simulink model "ex7"  (Simulink 6.0)
settings: Solver=ode45  StartTime=0.0  StopTime=50000  RelTol=1e-3
values from neighbouring files (symbols this model uses):
  SymbolRate = 1000    [ex11.m]    (also in ex2sim.m = 2; ex4sim.m = 2; ex7sim.m = 2)
libraries: commutil2 x4, commsink2 x2, commdigbbndpm2 x2, commchan2 x1, commrandsrc2 x1
settings Model: LastModifiedBy=lxy

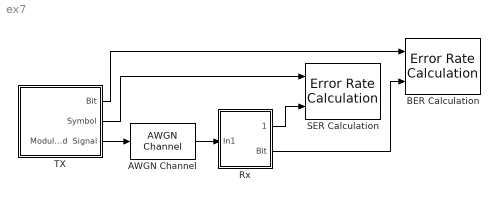
== system ex7 ==
  AWGN Channel : commchan2/AWGN Channel  seed=1111  noiseMode="Signal to noise ratio  (Es/No)"  EbNodB=10  EsNodB=SNR  SNRdB=10  bitsPerSym=1  Ps=1  Tsym=1/SymbolRate  variance=1
  BER Calculation : commsink2/Error Rate Calculation  N=0  st_delay=2*SymbolRate  cp_mode=Entire frame  subframe=[]  PMode=Workspace  WsName=BER  RsMode2=off  stop=on  numErr=100  maxBits=1e6
  Rx : Subsystem
  SER Calculation : commsink2/Error Rate Calculation  N=0  st_delay=SymbolRate  cp_mode=Entire frame  subframe=[]  PMode=Workspace  WsName=SER  RsMode2=off  stop=off  numErr=100  maxBits=1e6
  TX : Subsystem
  wires:
  TX/3(Modulated  Signal) -> AWGN Channel/1
  TX/2(Symbol) -> SER Calculation/1
  Rx/1(Symbol) -> SER Calculation/2
  Rx/2(Bit) -> BER Calculation/2
  TX/1(Bit) -> BER Calculation/1
  AWGN Channel/1 -> Rx/1(In1)

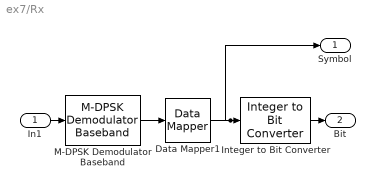
== system ex7/Rx ==
  In1 : Inport  Port=1  LatchInput=off
  Data Mapper1 : commutil2/Data Mapper  MapMode=Gray to Binary  M=4  MapVec=[0 1 3 2 7 6 4 5]
  Integer to Bit Converter : commutil2/Integer to Bit Converter  nbits=2
  M-DPSK Demodulator Baseband : commdigbbndpm2/M-DPSK Demodulator Baseband  M=4  OutType=Integer  Dec=Binary  Ph=0  numSamp=1
  Symbol : Outport
  Bit : Outport  Port=2
  wires:
  Integer to Bit Converter/1 -> Bit/1
  Data Mapper1/1 -> Symbol/1, Integer to Bit Converter/1
  In1/1 -> M-DPSK Demodulator Baseband/1
  M-DPSK Demodulator Baseband/1 -> Data Mapper1/1

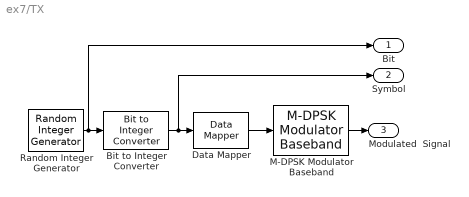
== system ex7/TX ==
  Bit to Integer Converter : commutil2/Bit to Integer Converter  nbits=2
  Data Mapper : commutil2/Data Mapper  MapMode=Binary to Gray  M=4  MapVec=[0 1 3 2 7 6 4 5]
  M-DPSK Modulator Baseband : commdigbbndpm2/M-DPSK Modulator Baseband  M=4  InType=Integer  Enc=Binary  Ph=0  numSamp=1
  Random Integer Generator : commrandsrc2/Random Integer Generator  mul=2  seed=37  Ts=1/(2*SymbolRate)  frameBased=on  sampPerFrame=2*SymbolRate  orient=off
  Bit : Outport
  Symbol : Outport  Port=2
  Modulated  Signal : Outport  Port=3
  wires:
  Data Mapper/1 -> M-DPSK Modulator Baseband/1
  M-DPSK Modulator Baseband/1 -> Modulated  Signal/1
  Random Integer Generator/1 -> Bit to Integer Converter/1, Bit/1
  Bit to Integer Converter/1 -> Data Mapper/1, Symbol/1
